simulink model "brake_system"  (R2022b)
settings: Solver=VariableStepAuto  StartTime=0.0  StopTime=10.0  RelTol=1e-3
model workspace (MAT data in the model file):
  driveLineGear = Simulink.Parameter
  driveLineGear.Value = 3.55
  driveLineGear.DataType = 'auto'
  driveLineGear.Complexity = 'real'
  driveLineGear.Dimensions = [1 1]
  maxBreakForce = Simulink.Parameter
  maxBreakForce.Value = 10000
  maxBreakForce.DataType = 'auto'
  maxBreakForce.Complexity = 'real'
  maxBreakForce.Dimensions = [1 1]
  regenFraction = Simulink.Parameter
  regenFraction.Value = 0.55
  regenFraction.DataType = 'auto'
  regenFraction.Complexity = 'real'
  regenFraction.Dimensions = [1 1]
  wheelRadius = Simulink.Parameter
  wheelRadius.Value = 0.35
  wheelRadius.DataType = 'auto'
  wheelRadius.Complexity = 'real'
  wheelRadius.Dimensions = [1 1]
libraries: simulink x1
settings Model: Creator=alexa  LastModifiedBy=alexa

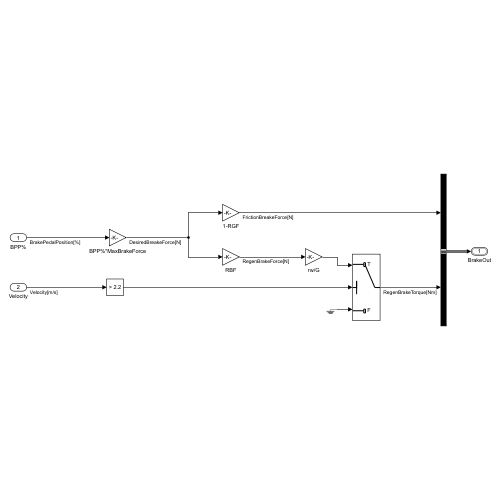
[thumbnail: Simulink's stored preview of the top-level diagram]
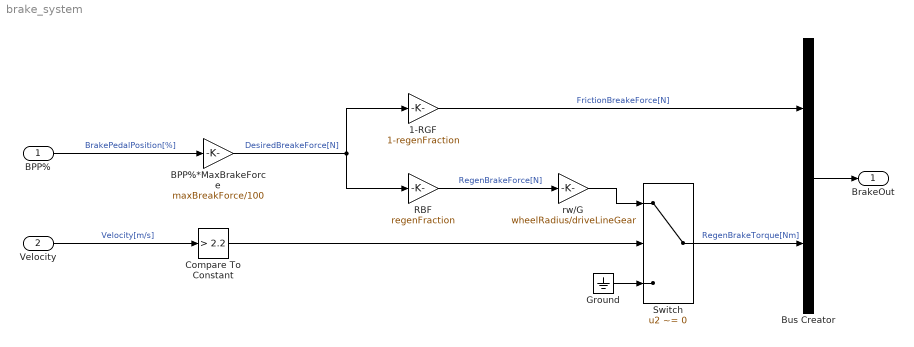
== system brake_system ==
  BPP% : Inport
  Velocity : Inport  Port=2
  1-RGF : Gain  Gain=1-regenFraction
  BPP%*MaxBrakeForce : Gain  Gain=maxBreakForce/100
  Bus Creator : BusCreator  Inputs=2
  Compare To Constant : simulink/Logic and Bit Operations/Compare To Constant  relop=>  const=2.2  OutDataTypeStr=boolean
  Ground : Ground
  RBF : Gain  Gain=regenFraction
  Switch : Switch  Criteria=u2 ~= 0  SaturateOnIntegerOverflow=off  InputSameDT=off
  rw/G : Gain  Gain=wheelRadius/driveLineGear
  BrakeOut : Outport  OutDataTypeStr=Bus: BusObject
  wires:
  BPP%/1 -> BPP%*MaxBrakeForce/1  "BrakePedalPosition[%]"
  BPP%*MaxBrakeForce/1 -> 1-RGF/1, RBF/1  "DesiredBreakeForce[N]"
  RBF/1 -> rw/G/1  "RegenBrakeForce[N]"
  Velocity/1 -> Compare To Constant/1  "Velocity[m/s]"
  rw/G/1 -> Switch/1
  Compare To Constant/1 -> Switch/2
  Ground/1 -> Switch/3
  1-RGF/1 -> Bus Creator/1  "FrictionBreakeForce[N]"
  Switch/1 -> Bus Creator/2  "RegenBrakeTorque[Nm]"
  Bus Creator/1 -> BrakeOut/1
